simulink model "float_sch_LocalMaxima_HardThreshold"  (R2020a)
settings: Solver=VariableStepAuto  StartTime=0  StopTime=30  RelTol=1e-3
model workspace (MAT data in the model file):
  a = 0
values from neighbouring files (symbols this model uses):
  fs = 30000    [float_sch_run_LocalMaxima_AdaptiveThreshold.m]    (also in float_sch_run_LocalMaxima_HardThreshold.m; float_sch_run_PTSD.m; float_sch_run_Sample_AdaptiveThreshold.m; float_sch_run_Sample_HardThreshold.m)
  refractory = 10^-3    (= 0.001)    [float_sch_run_LocalMaxima_AdaptiveThreshold.m]    (also in float_sch_run_LocalMaxima_HardThreshold.m; float_sch_run_PTSD.m; float_sch_run_Sample_AdaptiveThreshold.m; float_sch_run_Sample_HardThreshold.m)
  th = [-80:1:-40]    [float_sch_run_LocalMaxima_HardThreshold.m]    (also in float_sch_run_Sample_HardThreshold.m = [-80:10:-40])
libraries: dsparch4 x2, simulink x2, dspswit3 x1, hdlsllib x1
settings Model: SimulationMode=rapid-accelerator  ExtModeTrigDuration=100  Creator=sbuccelli  LastModifiedBy=diflo
settings DataIOCC: SaveOutput=off  StateSaveName=tmp_raccel_xout  SignalLoggingName=tmp_raccel_logsout
settings OptimizationCC: EfficientMapNaN2IntZero=off
settings HardwareCC: TargetBitPerPointer=64  TargetBitPerSizeT=64  TargetBitPerPtrDiffT=64  TargetLongLongMode=on  TargetIntDivRoundTo=Zero  TargetEndianess=LittleEndian  TargetWordSize=64  TargetHWDeviceType=MATLAB Host  ProdEqTarget=off
settings RTWCC: SystemTargetFile=raccel.tlc  TemplateMakefile=raccel_default_tmf  RTWVerbose=off  RTWUseSimCustomCode=on
settings CodeAppCC: GenerateComments=off  MaxIdLength=128  MangleLength=10
settings RaccelTargetCC: TargetLangStandard=C99 (ISO)  MultiInstanceERTCode=off  ENABLE_SLEXEC_SSBRIDGE=1  RTWCAPIParams=on  RTWCAPIRootIO=off

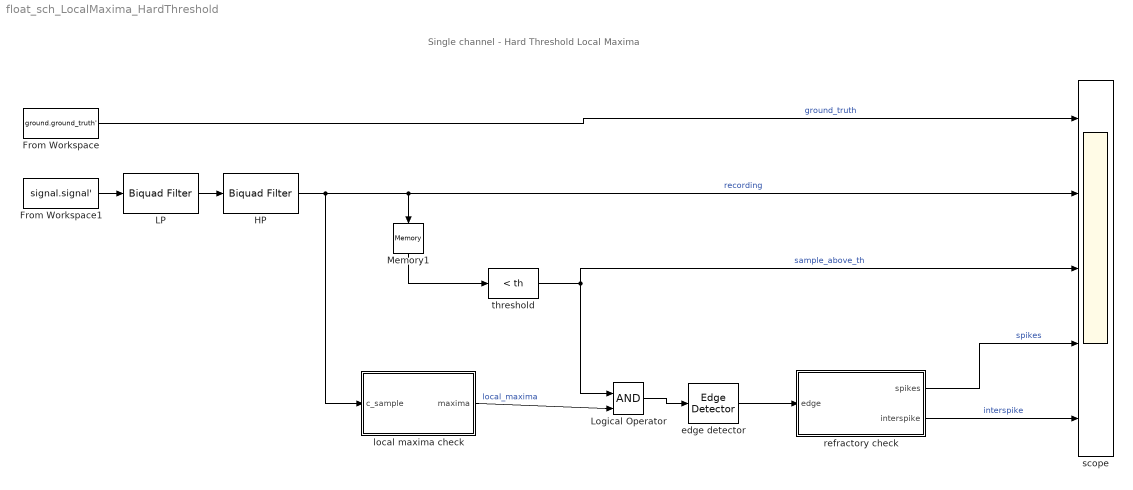
== system float_sch_LocalMaxima_HardThreshold ==
  note: Single channel - Hard Threshold Local Maxima
  From Workspace : FromWorkspace  VariableName=ground.ground_truth'  SampleTime=1/fs
  From Workspace1 : FromWorkspace  VariableName=signal.signal'  SampleTime=1/fs
  HP : dsparch4/Biquad Filter  Tag=BlockMethodSubSystem  FilterSource=Dialog parameters  CoeffSource=Specify via dialog  FilterObject=BQF  IIRFiltStruct=Direct form II  BiQuadCoeffs=[1 -2 1 1 -1.93529438685999167 0.93912079880642374;1 -1 0 1 -0.939062505817492399 0]  ScaleValues=[0.968603796416603768;0.969531252908746199;1]  IC=0  ICnum=0  ICden=0  a0Flag=Warning  optimizeScaleValues=on  ScaleValueMode=Specify via input port (g)  roundingMode=Floor  overflowMode=off  scaleValueFracLength=14  denProdOutputFracLength=30  denAccumFracLength=30  secondMemoryFracLength=15
  LP : dsparch4/Biquad Filter  Tag=BlockMethodSubSystem  FilterSource=Dialog parameters  CoeffSource=Specify via dialog  FilterObject=BQF  IIRFiltStruct=Direct form II  BiQuadCoeffs=[1 1 0 1 -0.509525449494428795 0]  ScaleValues=[0.245237275252785547;1]  IC=0  ICnum=0  ICden=0  a0Flag=Warning  optimizeScaleValues=on  ScaleValueMode=Specify via input port (g)  roundingMode=Floor  overflowMode=off  scaleValueFracLength=14  denProdOutputFracLength=30  denAccumFracLength=30  secondMemoryFracLength=15
  Logical Operator : Logic  IconShape=distinctive  AllPortsSameDT=off  OutDataTypeStr=boolean
  Memory1 : Memory  InheritSampleTime=on
  edge detector : dspswit3/Edge Detector  InputProcessing=Columns as channels (frame based)
      settings: SourceProductBaseCode=DS
  local maxima check : Subsystem
  refractory check : Subsystem
  scope : Scope  NumInputPorts=5
  threshold : simulink/Logic and Bit Operations/Compare To Constant  relop=<  const=th  OutDataTypeStr=boolean
  wires:
  refractory check/1(spikes) -> scope/4  "spikes"
  refractory check/2(interspike) -> scope/5  "interspike"
  edge detector/1 -> refractory check/1("edge ")
  threshold/1 -> Logical Operator/1, scope/3  "sample_above_th"
  Logical Operator/1 -> edge detector/1
  local maxima check/1(maxima) -> Logical Operator/2  "local_maxima"
  Memory1/1 -> threshold/1
  HP/1 -> local maxima check/1(c_sample), scope/2, Memory1/1  "recording"
  From Workspace1/1 -> LP/1
  LP/1 -> HP/1
  From Workspace/1 -> scope/1  "ground_truth"

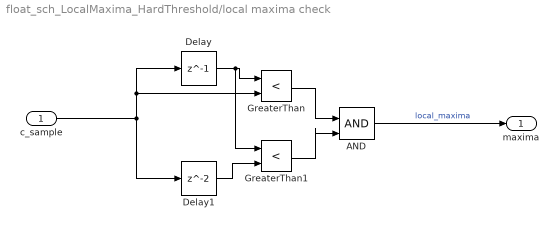
== system float_sch_LocalMaxima_HardThreshold/local maxima check ==
  c_sample : Inport
  AND : Logic  IconShape=distinctive  AllPortsSameDT=off  OutDataTypeStr=boolean
  Delay : Delay  DelayLength=1  SampleTime=1/30000
  Delay1 : Delay  SampleTime=1/30000
  GreaterThan : RelationalOperator  Operator=<  OutDataTypeStr=boolean  RndMeth=Simplest
  GreaterThan1 : RelationalOperator  Operator=<  OutDataTypeStr=boolean  RndMeth=Simplest
  maxima : Outport
  wires:
  Delay/1 -> GreaterThan1/1, GreaterThan/1
  c_sample/1 -> Delay/1, GreaterThan/2, Delay1/1
  GreaterThan/1 -> AND/1
  GreaterThan1/1 -> AND/2
  AND/1 -> maxima/1  "local_maxima"
  Delay1/1 -> GreaterThan1/2

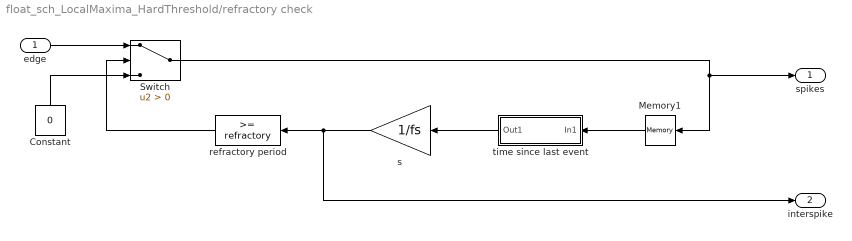
== system float_sch_LocalMaxima_HardThreshold/refractory check ==
  "edge " : Inport
  Constant : Constant  Value=0
  Memory1 : Memory  InheritSampleTime=on
  Switch : Switch  Criteria=u2 > Threshold
  refractory period : simulink/Logic and Bit Operations/Compare To Constant  relop=>=  const=refractory  OutDataTypeStr=boolean
  s : Gain  Gain=1/fs  ParamDataTypeStr=double
  time since last event : Subsystem
  spikes : Outport
  interspike : Outport  Port=2
  wires:
  "edge "/1 -> Switch/1
  Memory1/1 -> time since last event/1(In1)
  time since last event/1(Out1) -> s/1
  Constant/1 -> Switch/3
  s/1 -> refractory period/1, interspike/1
  Switch/1 -> spikes/1, Memory1/1
  refractory period/1 -> Switch/2

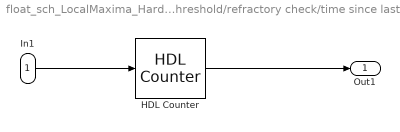
== system float_sch_LocalMaxima_HardThreshold/refractory check/time since last event ==
  In1 : Inport
  HDL Counter : hdlsllib/Sources/HDL Counter  CountType=Free running  CountInit=1  CountStep=1  CountMax=25  CountFromType=Initial value  CountFrom=1  CountResetPort=on  CountLoadPort=off  CountEnbPort=off  CountDirPort=off  CountDataType=Unsigned  CountWordLen=32  CountFracLen=0  CountSampTime=1
  Out1 : Outport
  wires:
  In1/1 -> HDL Counter/1
  HDL Counter/1 -> Out1/1
